simulink model "cascade_control"  (Simulink 8.1)
settings: Solver=ode45  StartTime=0.0  StopTime=inf  RelTol=1e-3
settings Model: Creator=eiseles  LastModifiedBy=eiseles
settings DataIOCC: SignalLoggingSaveFormat=Dataset
settings OptimizationCC: ExpressionDepthLimit=128
settings DebuggingCC: FcnCallInpInsideContextMsg=EnableAllAsError
settings GRTTargetCC: CombineOutputUpdateFcns=on  GRTInterface=off

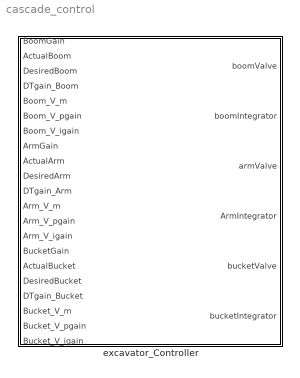
== system cascade_control ==
  excavator_Controller : Subsystem

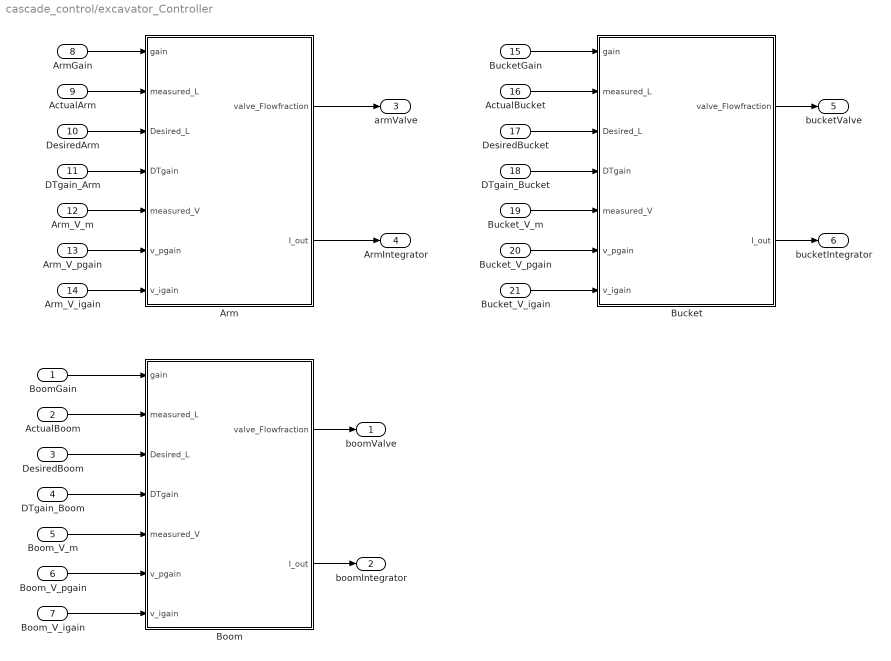
== system cascade_control/excavator_Controller ==
  BoomGain : Inport
  "ActualBoom " : Inport  Port=2
  DesiredBoom : Inport  Port=3
  DTgain_Boom : Inport  Port=4
  Boom_V_m : Inport  Port=5
  Boom_V_pgain : Inport  Port=6
  Boom_V_igain : Inport  Port=7
  ArmGain : Inport  Port=8
  ActualArm : Inport  Port=9
  DesiredArm : Inport  Port=10
  DTgain_Arm : Inport  Port=11
  Arm_V_m : Inport  Port=12
  Arm_V_pgain : Inport  Port=13
  Arm_V_igain : Inport  Port=14
  BucketGain : Inport  Port=15
  ActualBucket : Inport  Port=16
  DesiredBucket : Inport  Port=17
  DTgain_Bucket : Inport  Port=18
  Bucket_V_m : Inport  Port=19
  Bucket_V_pgain : Inport  Port=20
  Bucket_V_igain : Inport  Port=21
  "Arm " : Subsystem
  Boom : Subsystem
  Bucket : Subsystem
  boomValve : Outport
  boomIntegrator : Outport  Port=2
  armValve : Outport  Port=3
  ArmIntegrator : Outport  Port=4
  bucketValve : Outport  Port=5
  bucketIntegrator : Outport  Port=6
  wires:
  Bucket/1(valve_Flowfraction) -> bucketValve/1
  Bucket/2(I_out) -> bucketIntegrator/1
  DesiredBucket/1 -> Bucket/3(Desired_L)
  DTgain_Bucket/1 -> Bucket/4(DTgain)
  BucketGain/1 -> Bucket/1(gain)
  ActualBucket/1 -> Bucket/2(measured_L)
  Bucket_V_m/1 -> Bucket/5(measured_V)
  Bucket_V_pgain/1 -> Bucket/6(v_pgain)
  Bucket_V_igain/1 -> Bucket/7(v_igain)
  BoomGain/1 -> Boom/1(gain)
  "ActualBoom "/1 -> Boom/2(measured_L)
  DesiredBoom/1 -> Boom/3(Desired_L)
  DTgain_Boom/1 -> Boom/4(DTgain)
  Boom/1(valve_Flowfraction) -> boomValve/1
  Boom/2(I_out) -> boomIntegrator/1
  Boom_V_m/1 -> Boom/5(measured_V)
  Boom_V_pgain/1 -> Boom/6(v_pgain)
  Boom_V_igain/1 -> Boom/7(v_igain)
  ArmGain/1 -> "Arm "/1(gain)
  ActualArm/1 -> "Arm "/2(measured_L)
  DesiredArm/1 -> "Arm "/3(Desired_L)
  DTgain_Arm/1 -> "Arm "/4(DTgain)
  Arm_V_m/1 -> "Arm "/5(measured_V)
  Arm_V_pgain/1 -> "Arm "/6(v_pgain)
  Arm_V_igain/1 -> "Arm "/7(v_igain)
  "Arm "/1(valve_Flowfraction) -> armValve/1
  "Arm "/2(I_out) -> ArmIntegrator/1

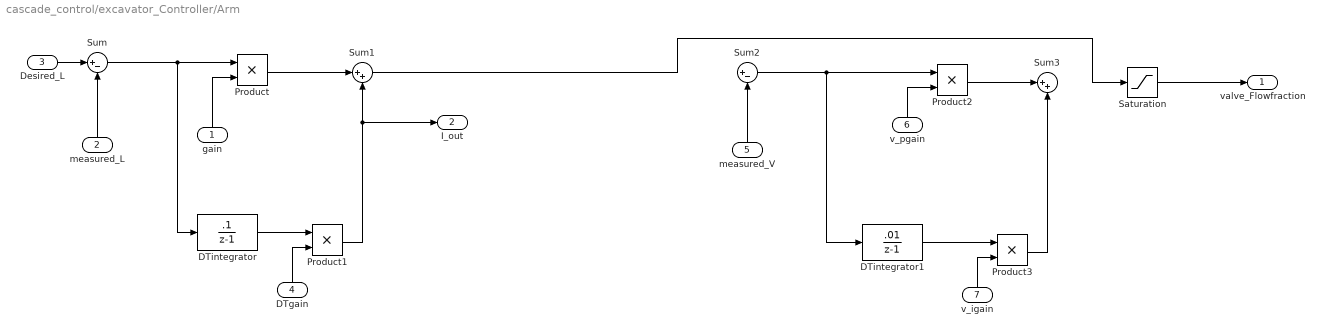
== system cascade_control/excavator_Controller/Arm  ==
  gain : Inport
  measured_L : Inport  Port=2
  Desired_L : Inport  Port=3
  DTgain : Inport  Port=4
  measured_V : Inport  Port=5
  v_pgain : Inport  Port=6
  v_igain : Inport  Port=7
  DTintegrator : DiscreteTransferFcn  Numerator=[.1]  Denominator=[1 -1]  SampleTime=.1  a0EqualsOne=on
  DTintegrator1 : DiscreteTransferFcn  Numerator=[.01]  Denominator=[1 -1]  SampleTime=.1  a0EqualsOne=on
  Product{,1..3} (4 alike) : Product
  Saturation : Saturate  UpperLimit=1  LowerLimit=-1
  Sum : Sum  Inputs=|+-
  Sum1 : Sum  Inputs=|++
  Sum2 : Sum  Inputs=|+-
  Sum3 : Sum  Inputs=|++
  valve_Flowfraction : Outport
  I_out : Outport  Port=2
  wires:
  measured_L/1 -> Sum/2
  Desired_L/1 -> Sum/1
  gain/1 -> Product/2
  Saturation/1 -> valve_Flowfraction/1
  Product/1 -> Sum1/1
  DTintegrator/1 -> Product1/1
  DTgain/1 -> Product1/2
  Product1/1 -> I_out/1, Sum1/2
  measured_V/1 -> Sum2/2
  Sum2/1 -> DTintegrator1/1, Product2/1
  v_pgain/1 -> Product2/2
  Product2/1 -> Sum3/1
  Product3/1 -> Sum3/2
  DTintegrator1/1 -> Product3/1
  v_igain/1 -> Product3/2
  Sum/1 -> DTintegrator/1, Product/1
  Sum1/1 -> Saturation/1

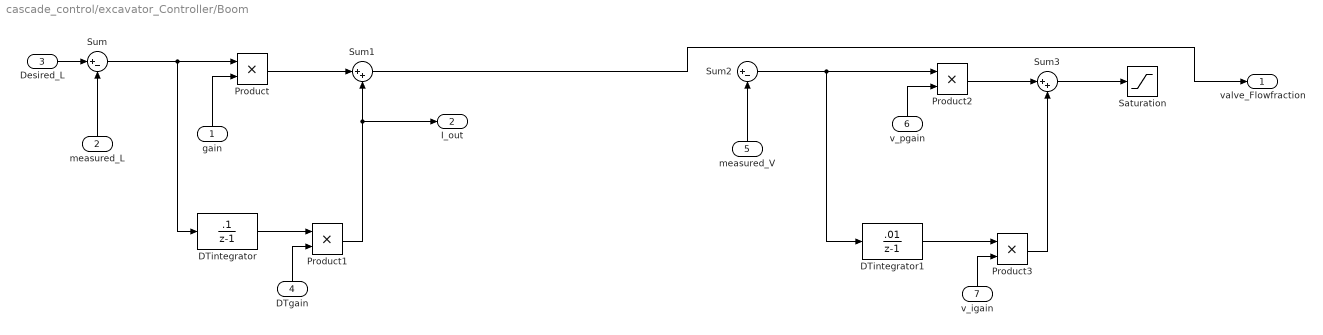
== system cascade_control/excavator_Controller/Boom ==
  gain : Inport
  measured_L : Inport  Port=2
  Desired_L : Inport  Port=3
  DTgain : Inport  Port=4
  measured_V : Inport  Port=5
  v_pgain : Inport  Port=6
  v_igain : Inport  Port=7
  DTintegrator : DiscreteTransferFcn  Numerator=[.1]  Denominator=[1 -1]  SampleTime=.1  a0EqualsOne=on
  DTintegrator1 : DiscreteTransferFcn  Numerator=[.01]  Denominator=[1 -1]  SampleTime=.1  a0EqualsOne=on
  Product{,1..3} (4 alike) : Product
  Saturation : Saturate  UpperLimit=1  LowerLimit=-1
  Sum : Sum  Inputs=|+-
  Sum1 : Sum  Inputs=|++
  Sum2 : Sum  Inputs=|+-
  Sum3 : Sum  Inputs=|++
  valve_Flowfraction : Outport
  I_out : Outport  Port=2
  wires:
  Sum/1 -> Product/1, DTintegrator/1
  v_igain/1 -> Product3/2
  DTintegrator1/1 -> Product3/1
  Product3/1 -> Sum3/2
  Sum3/1 -> Saturation/1
  Product2/1 -> Sum3/1
  v_pgain/1 -> Product2/2
  Sum2/1 -> Product2/1, DTintegrator1/1
  measured_V/1 -> Sum2/2
  Product1/1 -> Sum1/2, I_out/1
  DTgain/1 -> Product1/2
  DTintegrator/1 -> Product1/1
  Product/1 -> Sum1/1
  gain/1 -> Product/2
  Desired_L/1 -> Sum/1
  measured_L/1 -> Sum/2
  Sum1/1 -> valve_Flowfraction/1

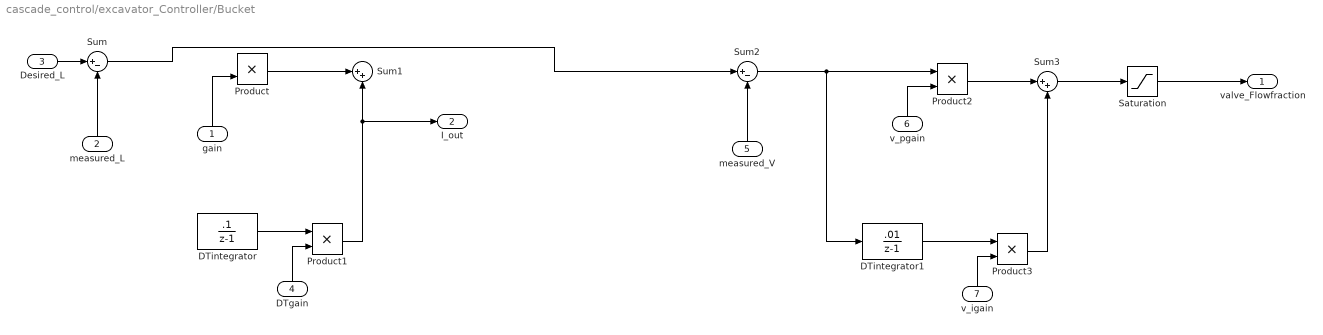
== system cascade_control/excavator_Controller/Bucket ==
  gain : Inport
  measured_L : Inport  Port=2
  Desired_L : Inport  Port=3
  DTgain : Inport  Port=4
  measured_V : Inport  Port=5
  v_pgain : Inport  Port=6
  v_igain : Inport  Port=7
  DTintegrator : DiscreteTransferFcn  Numerator=[.1]  Denominator=[1 -1]  SampleTime=.1  a0EqualsOne=on
  DTintegrator1 : DiscreteTransferFcn  Numerator=[.01]  Denominator=[1 -1]  SampleTime=.1  a0EqualsOne=on
  Product{,1..3} (4 alike) : Product
  Saturation : Saturate  UpperLimit=1  LowerLimit=-1
  Sum : Sum  Inputs=|+-
  Sum1 : Sum  Inputs=|++
  Sum2 : Sum  Inputs=|+-
  Sum3 : Sum  Inputs=|++
  valve_Flowfraction : Outport
  I_out : Outport  Port=2
  wires:
  measured_L/1 -> Sum/2
  Desired_L/1 -> Sum/1
  gain/1 -> Product/2
  Saturation/1 -> valve_Flowfraction/1
  Product/1 -> Sum1/1
  DTintegrator/1 -> Product1/1
  DTgain/1 -> Product1/2
  Product1/1 -> I_out/1, Sum1/2
  measured_V/1 -> Sum2/2
  Sum2/1 -> DTintegrator1/1, Product2/1
  v_pgain/1 -> Product2/2
  Product2/1 -> Sum3/1
  Sum3/1 -> Saturation/1
  Product3/1 -> Sum3/2
  DTintegrator1/1 -> Product3/1
  v_igain/1 -> Product3/2
  Sum/1 -> Sum2/1
